simulink model "Plant"  (R2024b)
settings: Solver=VariableStepAuto  StartTime=0.0  StopTime=8  RelTol=1e-3
undefined symbols (not defined in the file): c, d, eta, g, I, init_dq, init_q, J, Km, l, L, M, m, N, r, R, tau_m
settings Model: Creator=albin  LastModifiedBy=albin
settings DataIOCC: ReturnWorkspaceOutputs=off

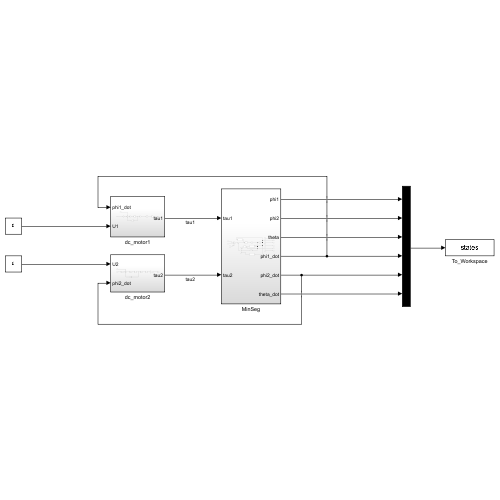
[thumbnail: Simulink's stored preview of the top-level diagram]
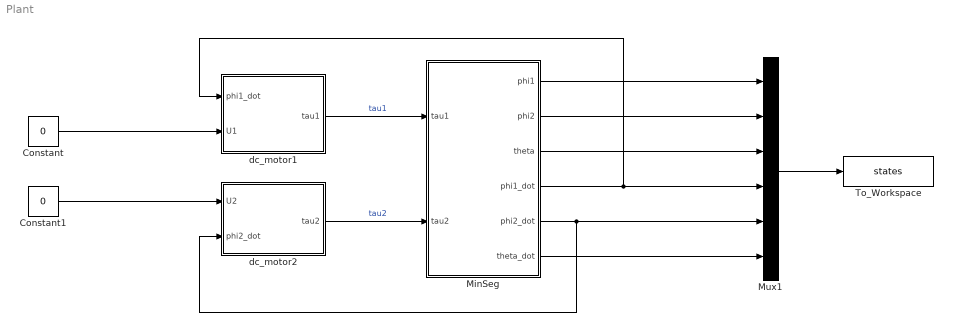
== system Plant ==
  Constant : Constant  Value=0
  Constant1 : Constant  Value=0
  MinSeg : Subsystem
  Mux1 : Mux  Inputs=6
  To_Workspace : ToWorkspace  VariableName=states  SaveFormat=Timeseries  SampleTime=-1
  dc_motor1 : Subsystem
  dc_motor2 : Subsystem
  wires:
  MinSeg/5(phi2_dot) -> Mux1/5, dc_motor2/2(phi2_dot)
  MinSeg/2(phi2) -> Mux1/2
  MinSeg/6(theta_dot) -> Mux1/6
  MinSeg/1(phi1) -> Mux1/1
  dc_motor2/1(tau2) -> MinSeg/2(tau2)  "tau2"
  MinSeg/4(phi1_dot) -> dc_motor1/1(phi1_dot), Mux1/4
  Constant/1 -> dc_motor1/2(U1)
  Constant1/1 -> dc_motor2/1(U2)
  Mux1/1 -> To_Workspace/1
  dc_motor1/1(tau1) -> MinSeg/1(tau1)  "tau1"
  MinSeg/3(theta) -> Mux1/3

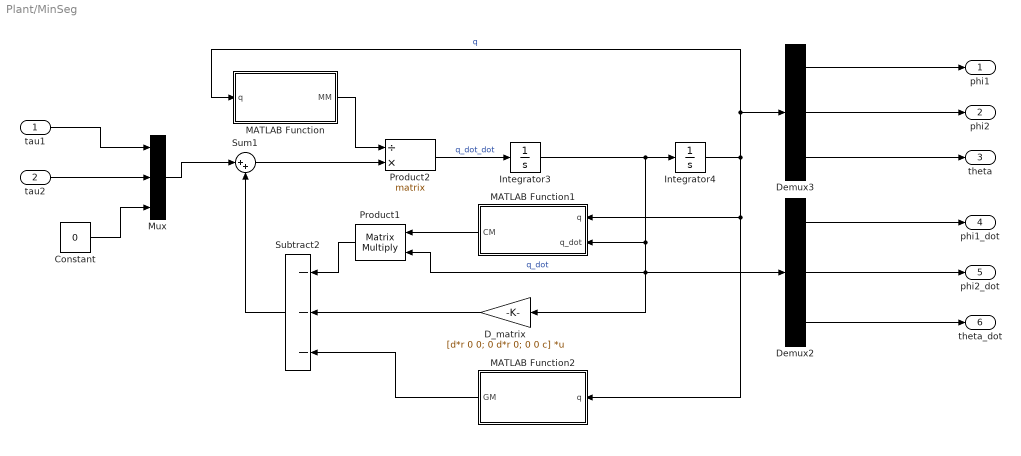
== system Plant/MinSeg ==
  tau1 : Inport
  tau2 : Inport  Port=2
  Constant : Constant  Value=0
  D_matrix : Gain  Gain=[d*r 0 0; 0 d*r 0; 0 0 c]  Multiplication=Matrix(K*u)
  Demux2 : Demux  Outputs=3
  Demux3 : Demux  Outputs=3
  Integrator3 : Integrator  InitialCondition=init_dq
  Integrator4 : Integrator  InitialCondition=init_q
  MATLAB Function : MATLAB Function  TreatAsAtomicUnit=on
  MATLAB Function1 : MATLAB Function  TreatAsAtomicUnit=on
  MATLAB Function2 : MATLAB Function  TreatAsAtomicUnit=on
  Mux : Mux  Inputs=3
  Product1 : Product  Multiplication=Matrix(*)
  Product2 : Product  Inputs=/*  Multiplication=Matrix(*)
  Subtract2 : Sum  Inputs=---
  Sum1 : Sum  Inputs=|++
  phi1 : Outport
  phi2 : Outport  Port=2
  theta : Outport  Port=3
  phi1_dot : Outport  Port=4
  phi2_dot : Outport  Port=5
  theta_dot : Outport  Port=6
  wires:
  Product2/1 -> Integrator3/1  "q_dot_dot"
  Mux/1 -> Sum1/1
  Constant/1 -> Mux/3
  Integrator4/1 -> MATLAB Function2/1(q), MATLAB Function1/1(q), Demux3/1, MATLAB Function/1(q)  "q"
  Demux3/2 -> phi2/1
  Demux2/1 -> phi1_dot/1
  MATLAB Function/1(MM) -> Product2/1
  Demux3/1 -> phi1/1
  Integrator3/1 -> MATLAB Function1/2(q_dot), D_matrix/1, Product1/2, Demux2/1, Integrator4/1  "q_dot"
  MATLAB Function2/1(GM) -> Subtract2/3
  Subtract2/1 -> Sum1/2
  MATLAB Function1/1(CM) -> Product1/1
  Product1/1 -> Subtract2/1
  Demux2/3 -> theta_dot/1
  Demux2/2 -> phi2_dot/1
  Demux3/3 -> theta/1
  Sum1/1 -> Product2/2
  D_matrix/1 -> Subtract2/2
  tau1/1 -> Mux/1
  tau2/1 -> Mux/2

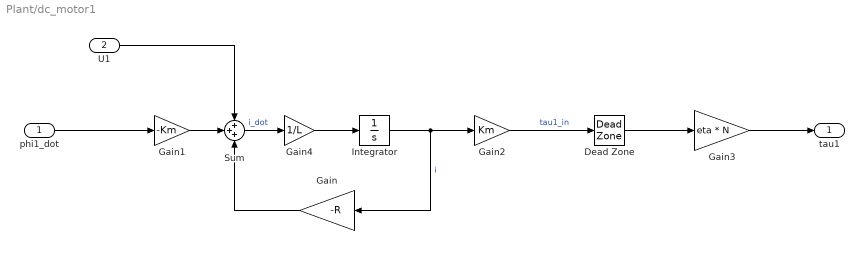
== system Plant/dc_motor1 ==
  phi1_dot : Inport
  U1 : Inport  Port=2
  Dead Zone : DeadZone  LowerValue=-tau_m  UpperValue=tau_m
  Gain : Gain  Gain=-R
  Gain1 : Gain  Gain=-Km
  Gain2 : Gain  Gain=Km
  Gain3 : Gain  Gain=eta * N
  Gain4 : Gain  Gain=1/L
  Integrator : Integrator
  Sum : Sum  Inputs=+++
  tau1 : Outport
  wires:
  Gain2/1 -> Dead Zone/1  "tau1_in"
  Integrator/1 -> Gain/1, Gain2/1  "i"
  Gain3/1 -> tau1/1
  Gain1/1 -> Sum/2
  Gain/1 -> Sum/3
  phi1_dot/1 -> Gain1/1
  Sum/1 -> Gain4/1  "i_dot"
  Gain4/1 -> Integrator/1
  U1/1 -> Sum/1
  Dead Zone/1 -> Gain3/1

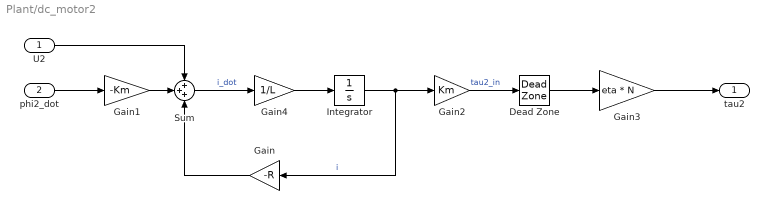
== system Plant/dc_motor2 ==
  U2 : Inport
  phi2_dot : Inport  Port=2
  Dead Zone : DeadZone  LowerValue=-tau_m  UpperValue=tau_m
  Gain : Gain  Gain=-R
  Gain1 : Gain  Gain=-Km
  Gain2 : Gain  Gain=Km
  Gain3 : Gain  Gain=eta * N
  Gain4 : Gain  Gain=1/L
  Integrator : Integrator
  Sum : Sum  Inputs=+++
  tau2 : Outport
  wires:
  Gain2/1 -> Dead Zone/1  "tau2_in"
  Integrator/1 -> Gain/1, Gain2/1  "i"
  Gain3/1 -> tau2/1
  U2/1 -> Sum/1
  Gain1/1 -> Sum/2
  Sum/1 -> Gain4/1  "i_dot"
  phi2_dot/1 -> Gain1/1
  Gain/1 -> Sum/3
  Dead Zone/1 -> Gain3/1
  Gain4/1 -> Integrator/1

== matlab function Plant/MinSeg/MATLAB Function1 ==
  data: q input; q_dot input; CM output; r parameter; M parameter; l parameter
function CM = C_matrix(q, q_dot, r, M, l)
    % initialize
    CM = zeros(3,3);

    % extract variables 
    theta = q(3);
    theta_dot = q_dot(3);

    % Calculate the elements of the C(q, q_dot) matrix
    CM(1,3) = -1/2*M*l*r*theta_dot*sin(theta);
    CM(2,3) = -1/2*M*l*r*theta_dot*sin(theta);
    CM(3,3) = -M*l*r*theta_dot*sin(theta);
end

== matlab function Plant/MinSeg/MATLAB Function ==
  data: q input; MM output; r parameter; m parameter; M parameter; l parameter; I parameter; J parameter
function MM = M_matrix(q, r, m, M, l, I, J)
    % initialize
    MM = zeros(3,3);
    
    % extract theta from q
    theta = q(3);

    % Calculate the elements of the M(q) matrix
    MM(1,1) = r^2*(1/4*M + m) + J;
    MM(1,2) = 1/4*M*r^2;
    MM(1,3) = r^2*(1/2*M + m) + J + 1/2*M*l*r*cos(theta);
    MM(2,1) = 1/4*M*r^2;
    MM(2,2) = r^2*(1/4*M + m) + J;
    MM(2,3) = r^2*(1/2*M + m) + J + 1/2*M*l*r*cos(theta);
    MM(3,1) = r^2*(1/2*M + m) + J + 1/2*M*l*r*cos(theta);
    MM(3,2) = r^2*(1/2*M + m) + J + 1/2*M*l*r*cos(theta);
    MM(3,3) = r^2*(M + 2*m) + 2*J + 2*M*l*r*cos(theta) + M*l^2 + I;
end

== matlab function Plant/MinSeg/MATLAB Function2 ==
  data: q input; GM output; g parameter; M parameter; l parameter
function GM = G_matrix(q, g, M, l)
    % extract theta from q
    theta = q(3);

    % Calculate the elements of the G(q) matrix
    GM = [0; 0; -M*g*l*sin(theta)];
end
